simulink model "Automatic_Turn_lights_with_Plant_model_in_continuous"  (R2026a)
settings: Solver=VariableStepAuto  StopTime=100
libraries: arduinolib x5, SignalEditorBlockLib x1
settings Model: SILPILSystemUnderTest=refmodels  Creator=irfan  LastModifiedBy=irfan

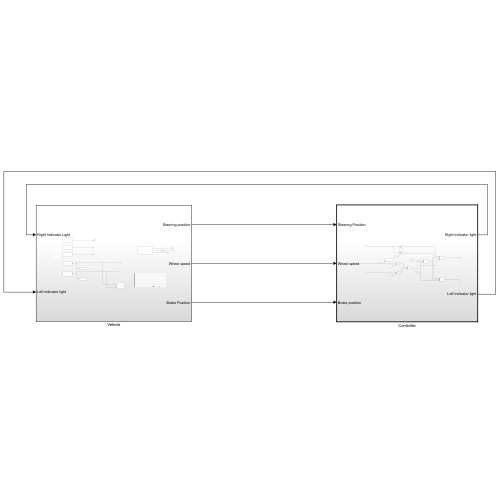
[thumbnail: Simulink's stored preview of the top-level diagram]
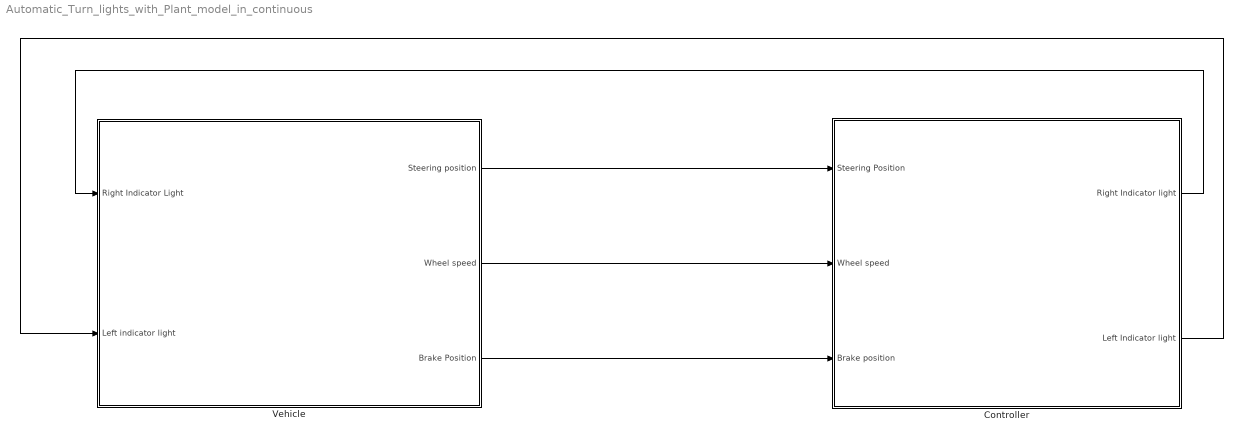
== system Automatic_Turn_lights_with_Plant_model_in_continuous ==
  Controller : Subsystem  TreatAsAtomicUnit=on
  Vehicle : Subsystem
  wires:
  Controller/1(Right Indicator light) -> Vehicle/1(Right Indicator Light)
  Controller/2(Left Indicator light) -> Vehicle/2(Left indicator light)
  Vehicle/1(Steering position) -> Controller/1(Steering Position)
  Vehicle/2(Wheel speed) -> Controller/2(Wheel speed)
  Vehicle/3(Brake Position) -> Controller/3(Brake position)

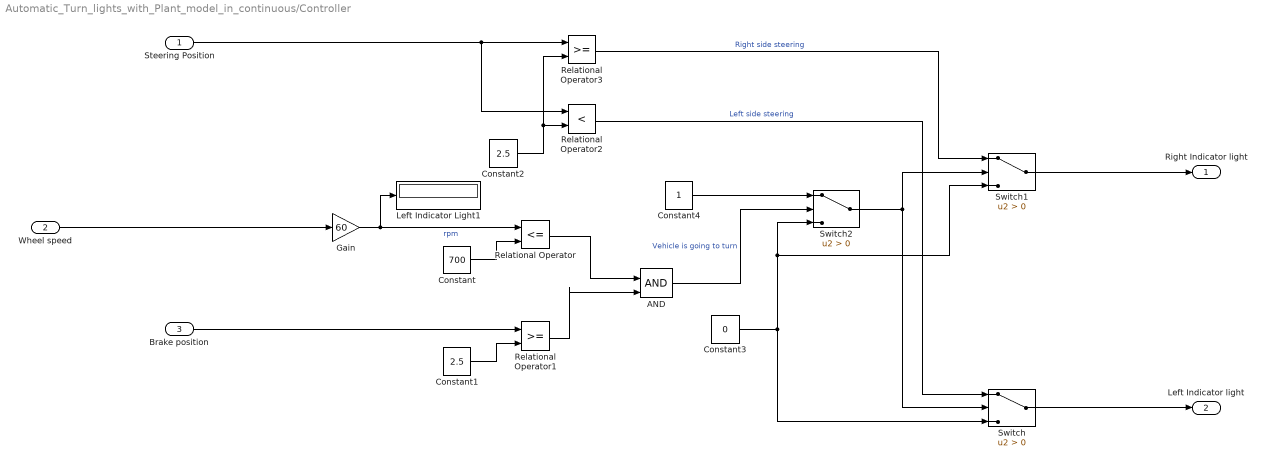
== system Automatic_Turn_lights_with_Plant_model_in_continuous/Controller ==
  Steering Position : Inport
  Wheel speed : Inport  Port=2
  Brake position : Inport  Port=3
  AND : Logic  IconShape=distinctive  AllPortsSameDT=off  OutDataTypeStr=boolean
  Constant : Constant  Value=700
  Constant1 : Constant  Value=2.5
  Constant2 : Constant  Value=2.5
  Constant3 : Constant  Value=0
  Constant4 : Constant
  Gain : Gain  Gain=60
  Left Indicator Light1 : Display
  Relational Operator : RelationalOperator  Operator=<=  OutDataTypeStr=boolean  RndMeth=Simplest  InputSameDT=off
  Relational Operator1 : RelationalOperator  OutDataTypeStr=boolean  RndMeth=Simplest  InputSameDT=off
  Relational Operator2 : RelationalOperator  Operator=<  OutDataTypeStr=boolean  RndMeth=Simplest  InputSameDT=off
  Relational Operator3 : RelationalOperator  OutDataTypeStr=boolean  RndMeth=Simplest  InputSameDT=off
  Switch : Switch  Criteria=u2 > Threshold  SaturateOnIntegerOverflow=off  InputSameDT=off
  Switch1 : Switch  Criteria=u2 > Threshold  SaturateOnIntegerOverflow=off  InputSameDT=off
  Switch2 : Switch  Criteria=u2 > Threshold  SaturateOnIntegerOverflow=off  InputSameDT=off
  Right Indicator light : Outport
  Left Indicator light : Outport  Port=2
  wires:
  Relational Operator2/1 -> Switch/1  "Left side steering"
  Relational Operator1/1 -> AND/2
  Steering Position/1 -> Relational Operator2/1, Relational Operator3/1
  Constant2/1 -> Relational Operator3/2, Relational Operator2/2
  AND/1 -> Switch2/2  "Vehicle is going to turn"
  Constant3/1 -> Switch2/3, Switch1/3, Switch/3
  Constant4/1 -> Switch2/1
  Constant1/1 -> Relational Operator1/2
  Switch2/1 -> Switch1/2, Switch/2
  Constant/1 -> Relational Operator/2
  Gain/1 -> Left Indicator Light1/1, Relational Operator/1  "rpm"
  Relational Operator3/1 -> Switch1/1  "Right side steering"
  Relational Operator/1 -> AND/1
  Switch/1 -> Left Indicator light/1
  Switch1/1 -> Right Indicator light/1
  Brake position/1 -> Relational Operator1/1
  Wheel speed/1 -> Gain/1

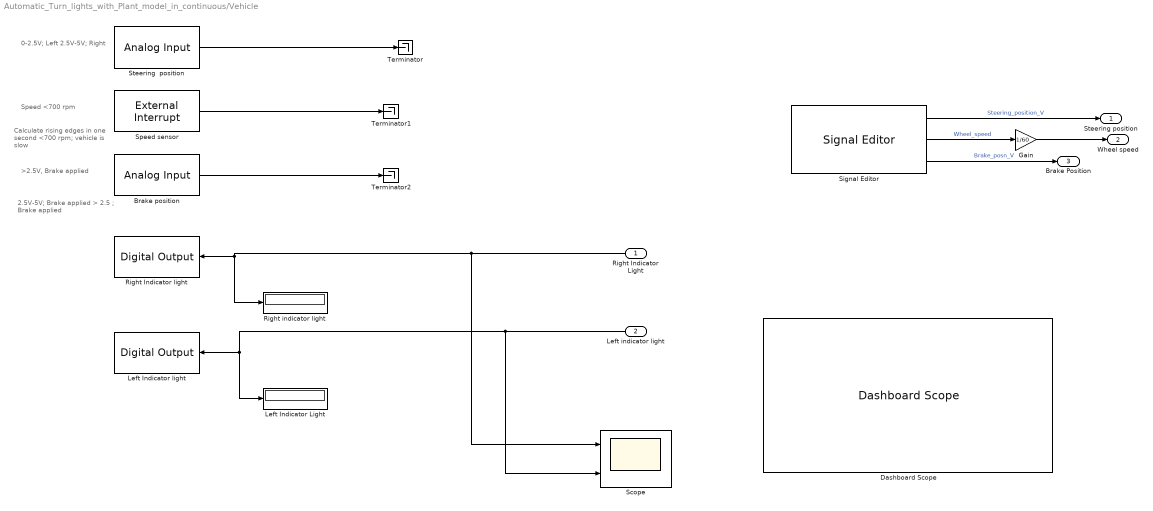
== system Automatic_Turn_lights_with_Plant_model_in_continuous/Vehicle ==
  note: 0-2.5V; Left
      | 2.5V-5V; Right
  note: Calculate rising edges
      | in one second
      | <700 rpm; vehicle is slow
  note: 2.5V-5V; Brake applied
      | > 2.5 ; Brake applied
  note: Speed <700 rpm
  note: >2.5V, Brake applied
  Right Indicator Light : Inport
  Left indicator light : Inport  Port=2
  Brake position : arduinolib/Analog Input  pinNumber=2  ReadResultsOnly=off  ConversionTriggerSource=Software  ExternalTriggerType=uint32( 0 )  OutputDataType=uint16  EnableConversionCompleteNotify=off  EnableOuputStatus=off  SampleTime=-1  blockPlatform=arduino
  Dashboard Scope : DashboardScope  TicksPosition=Inside  FontColor=[0.0, 0.0, 0.0]
  Gain : Gain  Gain=1/60
  Left Indicator Light : Display
  Left Indicator light : arduinolib/Digital Output  pinNumber=12  Direction=output  blockPlatform=arduino
  Right Indicator light : arduinolib/Digital Output  pinNumber=13  Direction=output  blockPlatform=arduino
  Right indicator light : Display
  Scope : Scope  NumInputPorts=2
      settings: ActiveDisplayYMinimum=-0.12499999999999997  ActiveDisplayYMaximum=1.125
  Signal Editor : SignalEditorBlockLib/Signal Editor  FileName=C:\Users\irfan\OneDrive\Documents\MATLAB\Blitz_Project\Signal_builder.mat  ActiveScenario=Test1  ActiveSignal=Steering_Position  IsBus=off  OutputBusObjectStr=Bus: BusObject  SampleTime=0  ZeroCross=off  OutputAfterFinalValue=Setting to zero  Unit=inherit  PreserveSignalName=on  ApplySigPropsToAllScenarios=on  ApplySigPropsToAllSignals=off  SignalPropertySource=Dialog parameters
  Speed sensor : arduinolib/External Interrupt  Pin=2  PullUp=off  Mode=RISING  InterruptSimulationInput=off
  Steering  position : arduinolib/Analog Input  pinNumber=1  ReadResultsOnly=off  ConversionTriggerSource=Software  ExternalTriggerType=uint32( 0 )  OutputDataType=uint16  EnableConversionCompleteNotify=off  EnableOuputStatus=off  SampleTime=-1  blockPlatform=arduino
  Terminator : Terminator
  Terminator1 : Terminator
  Terminator2 : Terminator
  Steering position : Outport
  Wheel speed : Outport  Port=2
  Brake Position : Outport  Port=3
  wires:
  Left indicator light/1 -> Scope/2, Left Indicator Light/1, Left Indicator light/1
  Right Indicator Light/1 -> Scope/1, Right indicator light/1, Right Indicator light/1
  Signal Editor/2 -> Gain/1  "Wheel_speed"
  Signal Editor/1 -> Steering position/1  "Steering_position_V"
  Gain/1 -> Wheel speed/1
  Signal Editor/3 -> Brake Position/1  "Brake_posn_V"
  Steering  position/1 -> Terminator/1
  Speed sensor/1 -> Terminator1/1
  Brake position/1 -> Terminator2/1
